simulink model "MotDynoReferenceApplication"  (R2026b)
settings: Solver=ode23tb  StartTime=0  StopTime=36  FixedStep=.001  RelTol=3e-2  EnableMultiTasking=on
libraries: simulink x2, autolibinverter x2, autolibpowerinfoutils x1, autolibpmsminterior x1, autolibfluxpmsm x1, autolibmappedmotor x1, autolibfluxmotorctrlr x1, autolibmotorctrlr x1
(part 4 of 7)

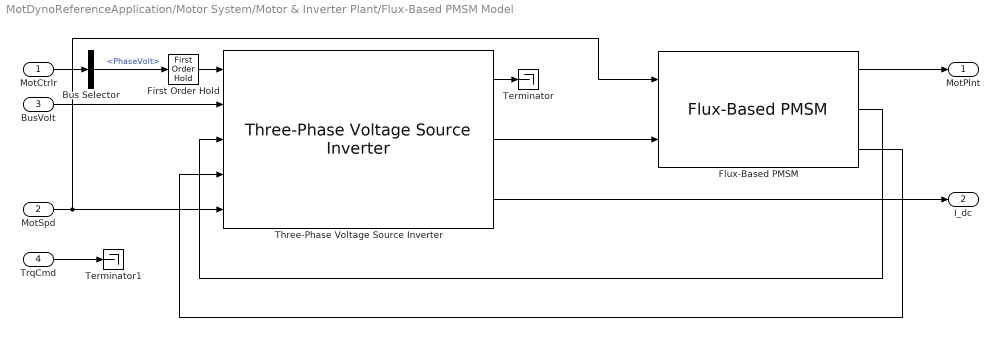
== system MotDynoReferenceApplication/Motor System/Motor & Inverter Plant/Flux-Based PMSM Model ==
  MotCtrlr : Inport
  MotSpd : Inport  Port=2
  BusVolt : Inport  Port=3
  TrqCmd : Inport  Port=4
  Bus Selector : BusSelector  OutputSignals=PhaseVolt
  First Order Hold : FirstOrderHold  ErrorTolerance=inf
  Flux-Based PMSM : autolibfluxpmsm/Flux-Based PMSM  VariantControl=Flux-Based PMSM Model  sim_type=Continuous  Ts=0.001  port_config=Speed  enable_hdl=off  flux_d=[-0.22607 -0.21687 -0.20768 -0.19848 -0.18928 -0.18009 -0.17089 -0.16169 -0.1525 -0.1433 -0.1341 -0.12491 -0.11571 -0.10651 -0.097316 -0.088119 -0.078922 -0.069725 -0.060529 -0.051332 -0.042135 -0.032938 -0.023742 -0.014545 -0.005348 0.0038488 0.013046 0.022242 0.031439 0.040636 0.049833 0.05903 0.068226 0.077423 0.08662 0.095817 0.10501 0.11421 0.12341 0.1326 0.1418 0.151 0.16019 0.16939 0.17859 0.18778 0.19698 0.20618 0.21537 0.22457]  n1=2  flux_q=[-0.4296 -0.41207 -0.39453 -0.377 -0.35947 -0.34193 -0.3244 -0.30686 -0.28933 -0.27179 -0.25426 -0.23672 -0.21919 -0.20165 -0.18412 -0.16659 -0.14905 -0.13152 -0.11398 -0.096447 -0.078913 -0.061378 -0.043844 -0.026309 -0.0087747 0.0087598 0.026294 0.043829 0.061363 0.078898 0.096433 0.11397 0.1315 0.14904 0.16657 0.18411 0.20164 0.21917 0.23671 0.25424 0.27178 0.28931 0.30685 0.32438 0.34192 0.35945 0.37699 0.39452 0.41205 0.42959]  n2=2  id=[-387.98 -381.91 -375.82 -369.71 -363.55 -357.36 -351.18 -345.07 -339.11 -333.43 -328.14 -323.36 -319.15 -315.54 -312.47 -309.87 -307.66 -305.82 -304.31 -303.09 -302.05 -301.17 -300.52 -300.13 -299.98 -299.99 -300.14 -300.54 -301.2 -302.07 -303.07 -304.29 -305.8 -307.66 -309.88 -312.48 -315.54 -319.13 -323.3 -328.03 -333.24 -338.83 -344.68 -350.68 -356.74 -362.82 -368.86 -374.87 -380.86 -386.83;-382.8 -375.91 -369.02 -362.13 -355.28 -348.49 -341.85 -335.42 -329.32 -323.64 -318.48 -313.91 -309.95 -306.58 -303.74 -301.34 -299.2 -297.4 -295.92 -294.7 -293.71 -292.88 -292.26 -291.86 -291.68 -291.68 -291.87 -292.27 -292.88 -293.7 -294.71 -295.92 -297.4 -299.21 -301.34 -303.75 -306.59 -309.95 -313.88 -318.42 -323.51 -329.11 -335.11 -341.43 -347.95 -354.61 -361.33 -368.08 -374.84 -381.6;-377.64 -369.91 -362.2 -354.54 -346.98 -339.59 -332.48 -325.75 -319.52 -313.88 -308.87 -304.51 -300.8 -297.66 -295.01 -292.74 -290.75 -289.02 -287.57 -286.37 -285.41 -284.64 -284.06 -283.66 -283.45 -283.46 -283.67 -284.06 -284.64 -285.4 -286.38 -287.58 -289.03 -290.75 -292.75 -295.03 -297.68 -300.82 -304.51 -308.85 -313.81 -319.38 -325.53 -332.15 -339.13 -346.37 -353.78 -361.28 -368.82 -376.38;-372.51 -363.91 -355.35 -346.89 -338.61 -330.62 -323.05 -316.03 -309.71 -304.17 -299.38 -295.27 -291.8 -288.86 -286.36 -284.22 -282.37 -280.75 -279.34 -278.17 -277.24 -276.53 -275.99 -275.59 -275.36 -275.37 -275.59 -275.98 -276.52 -277.24 -278.17 -279.35 -280.76 -282.38 -284.24 -286.39 -288.89 -291.83 -295.29 -299.39 -304.15 -309.64 -315.89 -322.8 -330.24 -338.07 -346.18 -354.45 -362.81 -371.19;-367.4 -357.89 -348.43 -339.12 -330.09 -321.49 -313.5 -306.27 -299.92 -294.6 -290.09 -286.26 -283.02 -280.26 -277.89 -275.88 -274.16 -272.64 -271.3 -270.15 -269.27 -268.61 -268.1 -267.72 -267.49 -267.48 -267.7 -268.09 -268.6 -269.26 -270.15 -271.31 -272.65 -274.17 -275.9 -277.92 -280.29 -283.06 -286.3 -290.12 -294.62 -299.92 -306.21 -313.34 -321.21 -329.64 -338.47 -347.55 -356.76 -366.03;-362.29 -351.79 -341.37 -331.16 -321.35 -312.14 -303.79 -296.51 -290.34 -285.25 -281.06 -277.53 -274.53 -271.94 -269.7 -267.8 -266.18 -264.76 -263.51 -262.43 -261.57 -260.91 -260.41 -260.06 -259.87 -259.86 -260.04 -260.4 -260.9 -261.57 -262.43 -263.51 -264.77 -266.2 -267.82 -269.72 -271.97 -274.56 -277.58 -281.11 -285.31 -290.39 -296.52 -303.72 -311.96 -320.99 -330.57 -340.51 -350.65 -360.85;-357.09 -345.52 -334.06 -322.9 -312.26 -302.51 -293.92 -286.75 -280.89 -276.17 -272.34 -269.11 -266.34 -263.93 -261.84 -260.03 -258.47 -257.11 -255.93 -254.92 -254.07 -253.4 -252.91 -252.58 -252.42 -252.41 -252.57 -252.9 -253.4 -254.07 -254.92 -255.94 -257.12 -258.48 -260.04 -261.85 -263.95 -266.37 -269.16 -272.4 -276.25 -280.98 -286.82 -293.94 -302.41 -312.01 -322.39 -333.25 -344.38 -355.59;-351.62 -338.93 -326.38 -314.19 -302.69 -292.47 -283.9 -277.04 -271.65 -267.37 -263.91 -260.99 -258.45 -256.22 -254.24 -252.5 -250.98 -249.66 -248.52 -247.55 -246.72 -246.04 -245.54 -245.23 -245.09 -245.08 -245.22 -245.54 -246.03 -246.72 -247.56 -248.53 -249.66 -250.99 -252.51 -254.26 -256.23 -258.47 -261.03 -263.98 -267.47 -271.76 -277.15 -283.97 -292.47 -302.55 -313.78 -325.63 -337.8 -350.1;-345.62 -331.79 -318.11 -304.8 -292.46 -281.98 -273.78 -267.54 -262.76 -258.98 -255.85 -253.17 -250.82 -248.73 -246.85 -245.15 -243.64 -242.34 -241.23 -240.3 -239.45 -238.77 -238.27 -237.96 -237.83 -237.83 -237.96 -238.27 -238.77 -239.45 -240.3 -241.23 -242.34 -243.65 -245.16 -246.86 -248.74 -250.84 -253.22 -255.93 -259.08 -262.89 -267.66 -273.86 -282.02 -292.43 -304.55 -317.43 -330.7 -344.13;-338.67 -323.78 -308.94 -294.27 -281.3 -271.17 -263.88 -258.49 -254.36 -251.02 -248.16 -245.63 -243.39 -241.39 -239.6 -237.91 -236.4 -235.1 -233.99 -233.05 -232.23 -231.56 -231.06 -230.74 -230.6 -230.6 -230.75 -231.07 -231.56 -232.23 -233.05 -234 -235.11 -236.41 -237.91 -239.6 -241.4 -243.41 -245.68 -248.23 -251.11 -254.48 -258.62 -263.96 -271.2 -281.36 -294.21 -308.38 -322.81 -337.31;-330.24 -314.48 -298.21 -282.34 -269.59 -260.87 ...(+15664 chars)]  iq=[-225.04 -214.57 -204 -193.21 -182.06 -170.46 -158.42 -146.03 -133.49 -121.08 -109.12 -97.871 -87.504 -78.066 -69.486 -61.607 -54.252 -47.304 -40.665 -34.237 -27.916 -21.645 -15.421 -9.2343 -3.0708 3.0879 9.2586 15.455 21.689 27.965 34.272 40.698 47.339 54.286 61.637 69.511 78.078 87.482 97.786 108.93 120.75 132.99 145.32 157.48 169.3 180.68 191.64 202.26 212.67 222.98;-238.44 -225.07 -211.66 -198.15 -184.5 -170.74 -156.97 -143.36 -130.12 -117.48 -105.65 -94.791 -84.983 -76.11 -68.008 -60.498 -53.351 -46.543 -40.002 -33.653 -27.424 -21.258 -15.143 -9.0662 -3.0111 3.0375 9.0946 15.174 21.29 27.455 33.69 40.037 46.575 53.383 60.526 68.04 76.139 84.995 94.767 105.55 117.27 129.75 142.8 156.19 169.72 183.22 196.61 209.88 223.05 236.17;-251.94 -235.62 -219.31 -203.03 -186.86 -170.93 -155.43 -140.61 -126.72 -113.92 -102.29 -91.821 -82.583 -74.238 -66.549 -59.333 -52.429 -45.781 -39.349 -33.085 -26.942 -20.879 -14.872 -8.9013 -2.9532 2.9869 8.9334 14.901 20.905 26.967 33.113 39.377 45.808 52.456 59.367 66.591 74.284 82.626 91.855 102.27 113.82 126.48 140.2 154.8 170.04 185.68 201.54 217.49 233.47 249.44;-265.66 -246.26 -226.92 -207.77 -188.99 -170.84 -153.63 -137.67 -123.24 -110.51 -99.246 -89.262 -80.48 -72.545 -65.185 -58.212 -51.512 -45.021 -38.706 -32.538 -26.485 -20.518 -14.611 -8.7432 -2.8983 2.9373 8.7783 14.641 20.542 26.506 32.558 38.725 45.041 51.538 58.249 65.232 72.61 80.559 89.329 99.291 110.5 123.14 137.41 153.16 170.1 187.93 206.33 225.08 243.98 262.93;-279.76 -257.03 -234.42 -212.19 -190.67 -170.26 -151.43 -134.55 -119.78 -107.39 -96.647 -87.18 -78.74 -71.078 -63.96 -57.178 -50.632 -44.275 -38.076 -32.011 -26.053 -20.178 -14.366 -8.5946 -2.8478 2.8893 8.6314 14.396 20.202 26.071 32.025 38.088 44.288 50.652 57.212 64.006 71.153 78.836 87.278 96.735 107.45 119.79 134.43 151.12 169.7 189.76 210.84 232.56 254.61 276.76;-294.31 -267.87 -241.66 -216.08 -191.65 -168.97 -148.7 -131.36 -116.78 -104.72 -94.502 -85.452 -77.274 -69.8 -62.852 -56.22 -49.79 -43.549 -37.463 -31.502 -25.64 -19.858 -14.135 -8.4555 -2.8016 2.8423 8.4923 14.166 19.881 25.657 31.512 37.471 43.556 49.799 56.238 62.9 69.876 77.378 85.568 94.6 104.82 116.87 131.36 148.52 168.6 190.92 214.85 239.81 265.33 291.03;-309.25 -278.64 -248.4 -219.14 -191.61 -166.84 -145.51 -128.05 -113.84 -102.28 -92.685 -83.953 -75.975 -68.645 -61.797 -55.273 -48.971 -42.847 -36.87 -31.011 -25.245 -19.551 -13.916 -8.3238 -2.7582 2.7971 8.3593 13.946 19.574 25.26 31.021 36.876 42.851 48.977 55.289 61.834 68.706 76.067 84.078 92.77 102.42 113.99 128.15 145.52 166.62 191.09 218.05 246.59 275.98 305.71;-324.3 -289.03 -254.29 -220.95 -190.17 -163.53 -141.79 -124.63 -110.95 -99.915 -90.677 -82.435 -74.75 -67.583 -60.831 -54.392 -48.186 -42.165 -36.293 -30.536 -24.861 -19.253 -13.704 -8.1966 -2.7167 2.753 8.23 13.732 19.276 24.877 30.547 36.301 42.171 48.194 54.407 60.857 67.621 74.797 82.493 90.83 100.09 111.14 124.77 141.92 163.57 189.89 220.08 252.53 286.28 320.58;-338.81 -298.48 -258.81 -220.9 -186.93 -158.91 -137.31 -121.02 -108.24 -97.825 -88.941 -80.978 -73.564 -66.574 -59.934 -53.567 -47.435 -41.501 -35.726 -30.07 -24.479 -18.957 -13.493 -8.0719 -2.6765 2.7092 8.1023 13.52 18.98 24.497 30.084 35.738 41.513 47.448 53.582 59.951 66.593 73.593 81.043 89.074 97.989 108.41 121.23 137.5 159.04 186.93 220.34 257.1 295.71 335.08;-351.58 -306.12 -261.13 -217.93 -180.97 -152.88 -132.61 -117.62 -105.89 -96.161 -87.587 -79.742 -72.444 -65.583 -59.063 -52.763 -46.704 -40.85 -35.158 -29.584 -24.089 -18.659 -13.284 -7.948 -2.6372 2.6649 7.9747 13.309 18.682 24.11 29.603 35.177 40.869 46.723 52.78 59.076 65.592 72.463 79.797 87.689 96.29 106.09 117.87 132.82 153.02 181.13 217.6 259.54 303.55 348.12;-360.76 -310.68 -259.27 -210.58 -172.63 -146.99 -128.89 -115.14 -104.12 -94.867 -86.478 -78.638 -71.374 -64.578 -58.133 -51.944 -45.979 -40.209 -34.597 -29.104 -23.699 -18.36 -13.073 -7.8236 -2.5977 2.6204 7.8466 13.096 18.384 23.723 29.129 34.622 40.235 46.004 51.966 58.146 64.581 71.372 78.652 ...(+14456 chars)]  preExtrapFlag=off  u1max=0.22457  u1min=-0.22607  u2max=0.42959  u2min=-0.4296  Rs=0.02  P=4  fluxdq0=[0 0]  theta_init=0  omega_init=0  mechanical=[0.0027, 4.924e-4, 0]  RefBlkName='autolibfluxpmsm/Flux-Based PMSM'  intPrec=23
  Terminator : Terminator
  Terminator1 : Terminator
  Three-Phase Voltage Source Inverter : autolibinverter/Three-Phase Voltage Source Inverter  InvrtrTmpInpEnbl=off  enable_hdl=off  model_type=Commanded phase voltage  fs=5000  w_eff_bp=[-1000 -500 0 500 1000]  n1=128  T_eff_bp=[-100 -50 0 50 100]*450  Temp_eff_bp=[213.15 293.15 373.15]  n2=128  ploss_table=0.98*ones(5,5)  ploss_table_3d=cat(3,0.95*[1 0.999 0.989 0.997 0.996;0.995 0.994 0.993 0.992 0.991;0.990 0.989 0.988 0.987 0.986;0.985 0.984 0.983 0.982 0.981;0.980 0.979 0.978 0.977 0.976],[1 0.999 0.989 0.997 0.996;0.995 0.994 0.993 0.992 0.991;0.990 0.989 0.988 0.987 0.986;0.985 0.984 0.983 0.982 0.981;0.980 0.979 0.978 0.977 0.976],0.92*[1 0.999 0.989 0.997 0.996;0.995 0.994 0.993 0.992 0.991;0.990 0.989 0.988 0.987 0.986;0.985 0.984 0.983 0.982 0.981;0.980 0.979 0.978 0.977 0.976])  preExtrapFlag=off  u1max=1000  u1min=-1000  u2max=200  u2min=-200  intPrec=23  RefBlkName='autolibmappedmotor/Mapped Motor'  CalLossMapData={}  CalLossWithTempMapData={}
  MotPlnt : Outport  VectorParamsAs1DForOutWhenUnconnected=off
  I_dc : Outport  Port=2  VectorParamsAs1DForOutWhenUnconnected=off
  wires:
  BusVolt/1 -> Three-Phase Voltage Source Inverter/2
  Flux-Based PMSM/1 -> MotPlnt/1
  MotSpd/1 -> Flux-Based PMSM/1, Three-Phase Voltage Source Inverter/5
  MotCtrlr/1 -> Bus Selector/1
  Flux-Based PMSM/3 -> Three-Phase Voltage Source Inverter/4
  Flux-Based PMSM/2 -> Three-Phase Voltage Source Inverter/3
  Three-Phase Voltage Source Inverter/1 -> Terminator/1
  Three-Phase Voltage Source Inverter/2 -> Flux-Based PMSM/2
  Three-Phase Voltage Source Inverter/3 -> I_dc/1
  Bus Selector/1 -> First Order Hold/1  "<PhaseVolt>"
  TrqCmd/1 -> Terminator1/1
  First Order Hold/1 -> Three-Phase Voltage Source Inverter/1
